simulink model "parabolic_interpolation"  (R2021a)
settings: Solver=FixedStepDiscrete  StartTime=0.0  StopTime=5  FixedStep=1  RelTol=1e-3
libraries: simulink x1
settings Model: Creator=manur  LastModifiedBy=manur

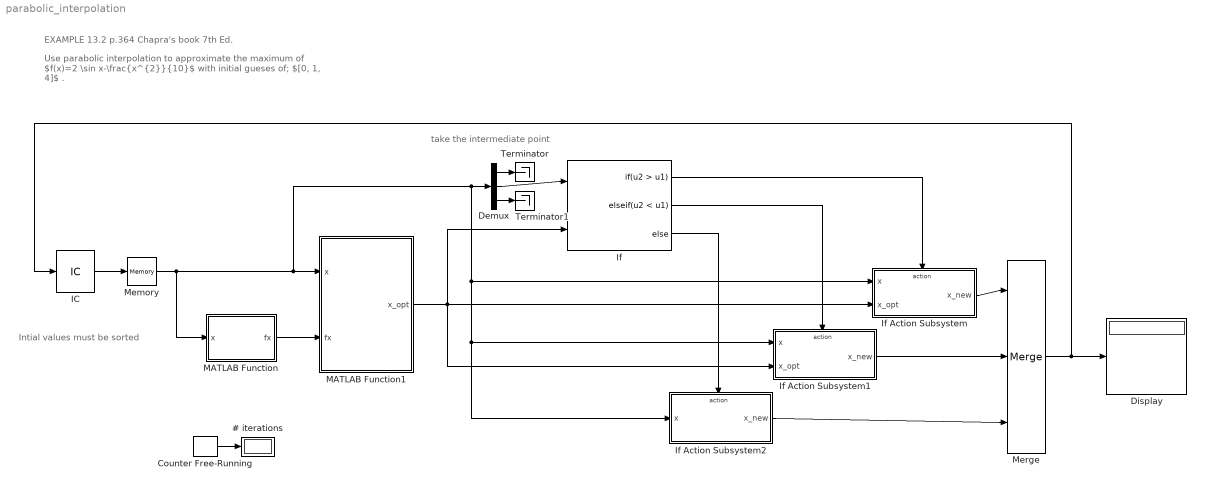
== system parabolic_interpolation ==
  note: EXAMPLE 13.2 p.364 Chapra's book 7th Ed.
  note: Use parabolic interpolation to approximate the maximum of
      | $f(x)=2 \sin x-\frac{x^{2}}{10}$
      | with initial gueses of; $[0, 1, 4]$ .
  note: Intial values must be sorted
  note: take the intermediate point
  # iterations : Display
  Counter Free-Running : simulink/Sources/Counter Free-Running  NumBits=16  tsamp=-1
  Demux : Demux  Outputs=3
  Display : Display
  IC : InitialCondition  Value=[0 1 4]
  If : If  NumInputs=2  IfExpression=u2 > u1  ElseIfExpressions=u2 < u1
  If Action Subsystem : Subsystem  TreatAsAtomicUnit=on
  If Action Subsystem1 : Subsystem  TreatAsAtomicUnit=on
  If Action Subsystem2 : Subsystem  TreatAsAtomicUnit=on
  MATLAB Function : MATLAB Function  TreatAsAtomicUnit=on
  MATLAB Function1 : MATLAB Function  TreatAsAtomicUnit=on
  Memory : Memory
  Merge : Merge  Inputs=3
  Terminator : Terminator
  Terminator1 : Terminator
  wires:
  Counter Free-Running/1 -> # iterations/1
  MATLAB Function/1(fx) -> MATLAB Function1/2(fx)
  Memory/1 -> Demux/1, If Action Subsystem2/1(x), If Action Subsystem1/1(x), If Action Subsystem/1(x), MATLAB Function1/1(x), MATLAB Function/1(x)
  MATLAB Function1/1(x_opt) -> If Action Subsystem1/2(x_opt), If Action Subsystem/2(x_opt), If/2
  If/1 -> If Action Subsystem/Action
  If/2 -> If Action Subsystem1/Action
  If/3 -> If Action Subsystem2/Action
  Demux/2 -> If/1
  Demux/1 -> Terminator/1
  Demux/3 -> Terminator1/1
  If Action Subsystem/1(x_new) -> Merge/1
  If Action Subsystem1/1(x_new) -> Merge/2
  If Action Subsystem2/1(x_new) -> Merge/3
  Merge/1 -> IC/1, Display/1
  IC/1 -> Memory/1

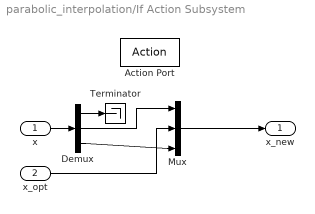
== system parabolic_interpolation/If Action Subsystem ==
  x : Inport
  x_opt : Inport  Port=2
  Action Port : ActionPort  ActionPortLabel=if(u2 > u1)
  Demux : Demux  Outputs=3
  Mux : Mux  Inputs=3
  Terminator : Terminator
  x_new : Outport
  wires:
  x/1 -> Demux/1
  Mux/1 -> x_new/1
  x_opt/1 -> Mux/2
  Demux/2 -> Mux/1
  Demux/3 -> Mux/3
  Demux/1 -> Terminator/1

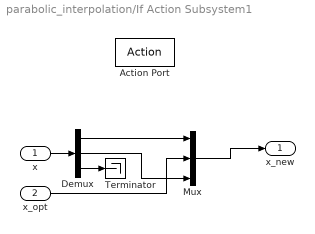
== system parabolic_interpolation/If Action Subsystem1 ==
  x : Inport
  x_opt : Inport  Port=2
  Action Port : ActionPort  ActionPortLabel=elseif(u2 < u1)
  Demux : Demux  Outputs=3
  Mux : Mux  Inputs=3
  Terminator : Terminator
  x_new : Outport
  wires:
  x/1 -> Demux/1
  Mux/1 -> x_new/1
  x_opt/1 -> Mux/2
  Demux/3 -> Terminator/1
  Demux/2 -> Mux/3
  Demux/1 -> Mux/1

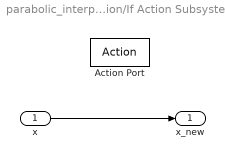
== system parabolic_interpolation/If Action Subsystem2 ==
  x : Inport
  Action Port : ActionPort  ActionPortLabel=else
  x_new : Outport
  wires:
  x/1 -> x_new/1

== matlab function parabolic_interpolation/MATLAB Function1 ==
  data: x input; x_opt output; fx input
function  x_opt = calc_x_opt(x, fx)

A = fx(1)*(x(2)^2-x(3)^2) + fx(2)*(x(3)^2-x(1)^2) + fx(3)*(x(1)^2-x(2)^2);
B = 2*fx(1)*(x(2)-x(3)) + 2*fx(2)*(x(3)-x(1)) + 2*fx(3)*(x(1)-x(2));

x_opt = A/B;

== matlab function parabolic_interpolation/MATLAB Function ==
  data: x input; fx output
function fx = f(x)

fx = 2*sin(x) - x.^2 / 10;
